simulink model "Crazyflie_angular_velocity_control_PID"  (R2020b)
settings: Solver=VariableStepAuto  StartTime=0.0  StopTime=5  RelTol=1e-3
libraries: pid_lib x4
settings Model: Creator=kt012  LastModifiedBy=kt012

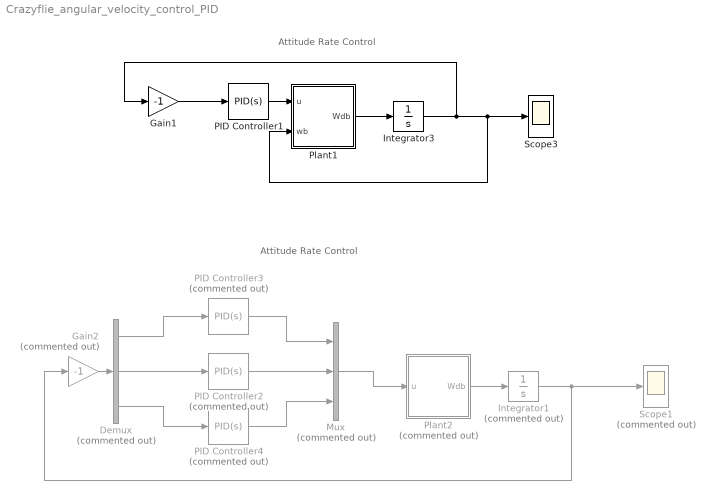
== system Crazyflie_angular_velocity_control_PID ==
  note: Attitude Rate Control
  note: Attitude Rate Control
  Demux : Demux  Commented=on  Outputs=3
  Gain1 : Gain  Gain=-1
  Gain2 : Gain  Commented=on  Gain=-1
  Integrator1 : Integrator  Commented=on  InitialCondition=[1 0 0];  ContinuousStateAttributes='Wb'
  Integrator3 : Integrator  InitialCondition=[1 0 0];  ContinuousStateAttributes='Wb'
  Mux : Mux  Commented=on  Inputs=3
  PID Controller1 : pid_lib/PID Controller  Controller=PID  Form=Parallel  TimeDomain=Continuous-time  UseExternalTs=off  SampleTime=-1  IntegratorMethod=Forward Euler  FilterMethod=Forward Euler  ControllerParametersSource=internal  P=2500  I=90  D=25  UseFilter=on  N=100  TunerSelectOption=Transfer Function Based (PID Tuner App)  InitialConditionSource=internal  InitialConditionForIntegrator=0  InitialConditionForFilter=0  DifferentiatorICPrevScaledInput=0  ExternalReset=none  TrackingMode=off  Kt=1  LimitOutput=off  SatLimitsSource=internal  UpperSaturationLimit=inf  LowerSaturationLimit=-inf  LinearizeAsGain=on  AntiWindupMode=none  Kb=1  POutMin=[]  POutMax=[]  IOutMin=[]  IOutMax=[]  DOutMin=[]  DOutMax=[]  NOutMin=[]  NOutMax=[]  SumOutMin=[]  SumOutMax=[]  SaturationOutMin=[]  SaturationOutMax=[]  PParamMin=[]  PParamMax=[]  IParamMin=[]  IParamMax=[]  DParamMin=[]  DParamMax=[]  NParamMin=[]  NParamMax=[]  KbParamMin=[]  KbParamMax=[]  KtParamMin=[]  KtParamMax=[]  KbOutMin=[]  KbOutMax=[]  KtOutMin=[]  KtOutMax=[]  IntegratorOutMin=[]  IntegratorOutMax=[]  FilterOutMin=[]  FilterOutMax=[]  SumI1OutMin=[]  SumI1OutMax=[]  SumI2OutMin=[]  SumI2OutMax=[]  SumI3OutMin=[]  SumI3OutMax=[]  SumI4OutMin=[]  SumI4OutMax=[]  SumDOutMin=[]  SumDOutMax=[]  DifferentiatorOutMin=[]  DifferentiatorOutMax=[]  FilterDiffOutCoefMin=[]  FilterDiffOutCoefMax=[]  ReciprocalOutMin=[]  ReciprocalOutMax=[]  SumDenOutMin=[]  SumDenOutMax=[]  SumNumOutMin=[]  SumNumOutMax=[]  DivideOutMin=[]  DivideOutMax=[]  UdiffTsProdOutMin=[]  UdiffTsProdOutMax=[]  NTsProdOutMin=[]  NTsProdOutMax=[]  UintegralTsProdOutMin=[]  UintegralTsProdOutMax=[]  UngainTsProdOutMin=[]  UngainTsProdOutMax=[]  IntegratorContinuousStateAttributes=''  IntegratorStateMustResolveToSignalObject=off  IntegratorRTWStateStorageClass=Auto  FilterContinuousStateAttributes=''  FilterStateMustResolveToSignalObject=off  FilterRTWStateStorageClass=Auto  ParallelPVariant=InternalParameters  IdealPVariant=Disabled  IVariant=InternalParameters  DVariant=InternalParameters  IntegratorVariant=Continuous  SatVariant=Disabled  AWVariant=Passthrough  PCopyVariant=Disabled  TRVariant=Disabled  FdbkBlocksVariant=Forward  IdealPFdbkVariant=Disabled  SatFdbkVariant=Disabled  DerivativeFilterVariant=ContFilter  NVariant=InternalParameters  NCopyVariant=Disabled  FilterICVariant=InternalICsFilter  IntegratorICVariant=InternalICs  ExternalResetVariant=Disabled  TRSumVariant=Passthrough  SumFdbkVariant=Disabled  SumVariant=Sum_PID  TsampFilterVariant=InternalTs  TsampNgainVariant=Passthrough  TsampIntegralVariant=Passthrough  ExternalSaturationOutDataTypeStr=Inherit: Same as second input
  PID Controller2 : pid_lib/PID Controller  Commented=on  Controller=PID  Form=Parallel  TimeDomain=Continuous-time  UseExternalTs=off  SampleTime=-1  IntegratorMethod=Forward Euler  FilterMethod=Forward Euler  ControllerParametersSource=internal  P=2500  I=90  D=25  UseFilter=on  N=100  TunerSelectOption=Transfer Function Based (PID Tuner App)  InitialConditionSource=internal  InitialConditionForIntegrator=0  InitialConditionForFilter=0  DifferentiatorICPrevScaledInput=0  ExternalReset=none  TrackingMode=off  Kt=1  LimitOutput=off  SatLimitsSource=internal  UpperSaturationLimit=inf  LowerSaturationLimit=-inf  LinearizeAsGain=on  AntiWindupMode=none  Kb=1  POutMin=[]  POutMax=[]  IOutMin=[]  IOutMax=[]  DOutMin=[]  DOutMax=[]  NOutMin=[]  NOutMax=[]  SumOutMin=[]  SumOutMax=[]  SaturationOutMin=[]  SaturationOutMax=[]  PParamMin=[]  PParamMax=[]  IParamMin=[]  IParamMax=[]  DParamMin=[]  DParamMax=[]  NParamMin=[]  NParamMax=[]  KbParamMin=[]  KbParamMax=[]  KtParamMin=[]  KtParamMax=[]  KbOutMin=[]  KbOutMax=[]  KtOutMin=[]  KtOutMax=[]  IntegratorOutMin=[]  IntegratorOutMax=[]  FilterOutMin=[]  FilterOutMax=[]  SumI1OutMin=[]  SumI1OutMax=[]  SumI2OutMin=[]  SumI2OutMax=[]  SumI3OutMin=[]  SumI3OutMax=[]  SumI4OutMin=[]  SumI4OutMax=[]  SumDOutMin=[]  SumDOutMax=[]  DifferentiatorOutMin=[]  DifferentiatorOutMax=[]  FilterDiffOutCoefMin=[]  FilterDiffOutCoefMax=[]  ReciprocalOutMin=[]  ReciprocalOutMax=[]  SumDenOutMin=[]  SumDenOutMax=[]  SumNumOutMin=[]  SumNumOutMax=[]  DivideOutMin=[]  DivideOutMax=[]  UdiffTsProdOutMin=[]  UdiffTsProdOutMax=[]  NTsProdOutMin=[]  NTsProdOutMax=[]  UintegralTsProdOutMin=[]  UintegralTsProdOutMax=[]  UngainTsProdOutMin=[]  UngainTsProdOutMax=[]  IntegratorContinuousStateAttributes=''  IntegratorStateMustResolveToSignalObject=off  IntegratorRTWStateStorageClass=Auto  FilterContinuousStateAttributes=''  FilterStateMustResolveToSignalObject=off  FilterRTWStateStorageClass=Auto  ParallelPVariant=InternalParameters  IdealPVariant=Disabled  IVariant=InternalParameters  DVariant=InternalParameters  IntegratorVariant=Continuous  SatVariant=Disabled  AWVariant=Passthrough  PCopyVariant=Disabled  TRVariant=Disabled  FdbkBlocksVariant=Forward  IdealPFdbkVariant=Disabled  SatFdbkVariant=Disabled  DerivativeFilterVariant=ContFilter  NVariant=InternalParameters  NCopyVariant=Disabled  FilterICVariant=InternalICsFilter  IntegratorICVariant=InternalICs  ExternalResetVariant=Disabled  TRSumVariant=Passthrough  SumFdbkVariant=Disabled  SumVariant=Sum_PID  TsampFilterVariant=InternalTs  TsampNgainVariant=Passthrough  TsampIntegralVariant=Passthrough  ExternalSaturationOutDataTypeStr=Inherit: Same as second input
  PID Controller3 : pid_lib/PID Controller  Commented=on  Controller=PID  Form=Parallel  TimeDomain=Continuous-time  UseExternalTs=off  SampleTime=-1  IntegratorMethod=Forward Euler  FilterMethod=Forward Euler  ControllerParametersSource=internal  P=1250  I=2500  D=20  UseFilter=on  N=90.5133762745109  TunerSelectOption=Transfer Function Based (PID Tuner App)  InitialConditionSource=internal  InitialConditionForIntegrator=0  InitialConditionForFilter=0  DifferentiatorICPrevScaledInput=0  ExternalReset=none  TrackingMode=off  Kt=1  LimitOutput=off  SatLimitsSource=internal  UpperSaturationLimit=inf  LowerSaturationLimit=-inf  LinearizeAsGain=on  AntiWindupMode=none  Kb=1  POutMin=[]  POutMax=[]  IOutMin=[]  IOutMax=[]  DOutMin=[]  DOutMax=[]  NOutMin=[]  NOutMax=[]  SumOutMin=[]  SumOutMax=[]  SaturationOutMin=[]  SaturationOutMax=[]  PParamMin=[]  PParamMax=[]  IParamMin=[]  IParamMax=[]  DParamMin=[]  DParamMax=[]  NParamMin=[]  NParamMax=[]  KbParamMin=[]  KbParamMax=[]  KtParamMin=[]  KtParamMax=[]  KbOutMin=[]  KbOutMax=[]  KtOutMin=[]  KtOutMax=[]  IntegratorOutMin=[]  IntegratorOutMax=[]  FilterOutMin=[]  FilterOutMax=[]  SumI1OutMin=[]  SumI1OutMax=[]  SumI2OutMin=[]  SumI2OutMax=[]  SumI3OutMin=[]  SumI3OutMax=[]  SumI4OutMin=[]  SumI4OutMax=[]  SumDOutMin=[]  SumDOutMax=[]  DifferentiatorOutMin=[]  DifferentiatorOutMax=[]  FilterDiffOutCoefMin=[]  FilterDiffOutCoefMax=[]  ReciprocalOutMin=[]  ReciprocalOutMax=[]  SumDenOutMin=[]  SumDenOutMax=[]  SumNumOutMin=[]  SumNumOutMax=[]  DivideOutMin=[]  DivideOutMax=[]  UdiffTsProdOutMin=[]  UdiffTsProdOutMax=[]  NTsProdOutMin=[]  NTsProdOutMax=[]  UintegralTsProdOutMin=[]  UintegralTsProdOutMax=[]  UngainTsProdOutMin=[]  UngainTsProdOutMax=[]  IntegratorContinuousStateAttributes=''  IntegratorStateMustResolveToSignalObject=off  IntegratorRTWStateStorageClass=Auto  FilterContinuousStateAttributes=''  FilterStateMustResolveToSignalObject=off  FilterRTWStateStorageClass=Auto  ParallelPVariant=InternalParameters  IdealPVariant=Disabled  IVariant=InternalParameters  DVariant=InternalParameters  IntegratorVariant=Continuous  SatVariant=Disabled  AWVariant=Passthrough  PCopyVariant=Disabled  TRVariant=Disabled  FdbkBlocksVariant=Forward  IdealPFdbkVariant=Disabled  SatFdbkVariant=Disabled  DerivativeFilterVariant=ContFilter  NVariant=InternalParameters  NCopyVariant=Disabled  FilterICVariant=InternalICsFilter  IntegratorICVariant=InternalICs  ExternalResetVariant=Disabled  TRSumVariant=Passthrough  SumFdbkVariant=Disabled  SumVariant=Sum_PID  TsampFilterVariant=InternalTs  TsampNgainVariant=Passthrough  TsampIntegralVariant=Passthrough  ExternalSaturationOutDataTypeStr=Inherit: Same as second input
  PID Controller4 : pid_lib/PID Controller  Commented=on  Controller=PID  Form=Parallel  TimeDomain=Continuous-time  UseExternalTs=off  SampleTime=-1  IntegratorMethod=Forward Euler  FilterMethod=Forward Euler  ControllerParametersSource=internal  P=2500  I=90  D=25  UseFilter=on  N=100  TunerSelectOption=Transfer Function Based (PID Tuner App)  InitialConditionSource=internal  InitialConditionForIntegrator=0  InitialConditionForFilter=0  DifferentiatorICPrevScaledInput=0  ExternalReset=none  TrackingMode=off  Kt=1  LimitOutput=off  SatLimitsSource=internal  UpperSaturationLimit=inf  LowerSaturationLimit=-inf  LinearizeAsGain=on  AntiWindupMode=none  Kb=1  POutMin=[]  POutMax=[]  IOutMin=[]  IOutMax=[]  DOutMin=[]  DOutMax=[]  NOutMin=[]  NOutMax=[]  SumOutMin=[]  SumOutMax=[]  SaturationOutMin=[]  SaturationOutMax=[]  PParamMin=[]  PParamMax=[]  IParamMin=[]  IParamMax=[]  DParamMin=[]  DParamMax=[]  NParamMin=[]  NParamMax=[]  KbParamMin=[]  KbParamMax=[]  KtParamMin=[]  KtParamMax=[]  KbOutMin=[]  KbOutMax=[]  KtOutMin=[]  KtOutMax=[]  IntegratorOutMin=[]  IntegratorOutMax=[]  FilterOutMin=[]  FilterOutMax=[]  SumI1OutMin=[]  SumI1OutMax=[]  SumI2OutMin=[]  SumI2OutMax=[]  SumI3OutMin=[]  SumI3OutMax=[]  SumI4OutMin=[]  SumI4OutMax=[]  SumDOutMin=[]  SumDOutMax=[]  DifferentiatorOutMin=[]  DifferentiatorOutMax=[]  FilterDiffOutCoefMin=[]  FilterDiffOutCoefMax=[]  ReciprocalOutMin=[]  ReciprocalOutMax=[]  SumDenOutMin=[]  SumDenOutMax=[]  SumNumOutMin=[]  SumNumOutMax=[]  DivideOutMin=[]  DivideOutMax=[]  UdiffTsProdOutMin=[]  UdiffTsProdOutMax=[]  NTsProdOutMin=[]  NTsProdOutMax=[]  UintegralTsProdOutMin=[]  UintegralTsProdOutMax=[]  UngainTsProdOutMin=[]  UngainTsProdOutMax=[]  IntegratorContinuousStateAttributes=''  IntegratorStateMustResolveToSignalObject=off  IntegratorRTWStateStorageClass=Auto  FilterContinuousStateAttributes=''  FilterStateMustResolveToSignalObject=off  FilterRTWStateStorageClass=Auto  ParallelPVariant=InternalParameters  IdealPVariant=Disabled  IVariant=InternalParameters  DVariant=InternalParameters  IntegratorVariant=Continuous  SatVariant=Disabled  AWVariant=Passthrough  PCopyVariant=Disabled  TRVariant=Disabled  FdbkBlocksVariant=Forward  IdealPFdbkVariant=Disabled  SatFdbkVariant=Disabled  DerivativeFilterVariant=ContFilter  NVariant=InternalParameters  NCopyVariant=Disabled  FilterICVariant=InternalICsFilter  IntegratorICVariant=InternalICs  ExternalResetVariant=Disabled  TRSumVariant=Passthrough  SumFdbkVariant=Disabled  SumVariant=Sum_PID  TsampFilterVariant=InternalTs  TsampNgainVariant=Passthrough  TsampIntegralVariant=Passthrough  ExternalSaturationOutDataTypeStr=Inherit: Same as second input
  Plant1 : Subsystem
  Plant2 : Subsystem  Commented=on
  Scope1 : Scope  Commented=on
  Scope3 : Scope
  wires:
  PID Controller1/1 -> Plant1/1(u)
  Plant1/1(Wdb) -> Integrator3/1
  Gain1/1 -> PID Controller1/1
  Integrator3/1 -> Gain1/1, Plant1/2(wb), Scope3/1
  PID Controller2/1 -> Mux/2
  Integrator1/1 -> Gain2/1, Scope1/1
  Gain2/1 -> Demux/1
  Plant2/1(Wdb) -> Integrator1/1
  Demux/1 -> PID Controller3/1
  Demux/2 -> PID Controller2/1
  Demux/3 -> PID Controller4/1
  PID Controller4/1 -> Mux/3
  PID Controller3/1 -> Mux/1
  Mux/1 -> Plant2/1(u)

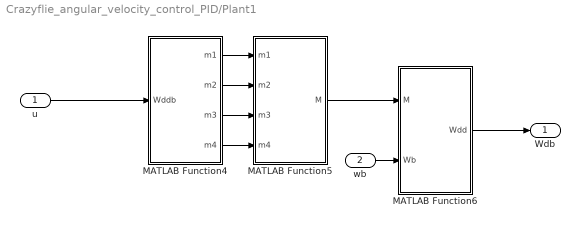
== system Crazyflie_angular_velocity_control_PID/Plant1 ==
  u : Inport
  wb : Inport  Port=2
  MATLAB Function4 : MATLAB Function  TreatAsAtomicUnit=on
  MATLAB Function5 : MATLAB Function  TreatAsAtomicUnit=on
  MATLAB Function6 : MATLAB Function  TreatAsAtomicUnit=on
  Wdb : Outport
  wires:
  wb/1 -> MATLAB Function6/2(Wb)
  MATLAB Function5/1(M) -> MATLAB Function6/1(M)
  MATLAB Function6/1(Wdd) -> Wdb/1
  MATLAB Function4/3(m3) -> MATLAB Function5/3(m3)
  MATLAB Function4/2(m2) -> MATLAB Function5/2(m2)
  MATLAB Function4/4(m4) -> MATLAB Function5/4(m4)
  u/1 -> MATLAB Function4/1(Wddb)
  MATLAB Function4/1(m1) -> MATLAB Function5/1(m1)

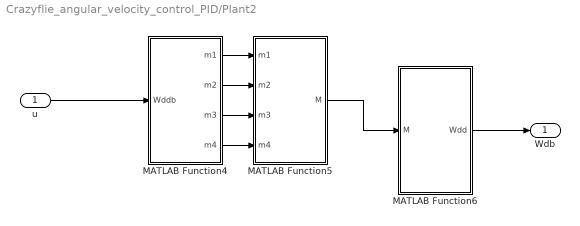
== system Crazyflie_angular_velocity_control_PID/Plant2 ==
  u : Inport
  MATLAB Function4 : MATLAB Function  TreatAsAtomicUnit=on
  MATLAB Function5 : MATLAB Function  TreatAsAtomicUnit=on
  MATLAB Function6 : MATLAB Function  TreatAsAtomicUnit=on
  Wdb : Outport
  wires:
  MATLAB Function5/1(M) -> MATLAB Function6/1(M)
  MATLAB Function6/1(Wdd) -> Wdb/1
  MATLAB Function4/3(m3) -> MATLAB Function5/3(m3)
  MATLAB Function4/2(m2) -> MATLAB Function5/2(m2)
  MATLAB Function4/4(m4) -> MATLAB Function5/4(m4)
  u/1 -> MATLAB Function4/1(Wddb)
  MATLAB Function4/1(m1) -> MATLAB Function5/1(m1)

== matlab function Crazyflie_angular_velocity_control_PID/Plant1/MATLAB Function4 ==
  data: Wddb input; m1 output; m2 output; m3 output; m4 output
function [m1, m2, m3, m4]= fcn(Wddb)

% F [16bit] Wddb [16bit]

r = min(max(-32000, Wddb(1)), 32000)/2;
p = min(max(-32000, Wddb(2)), 32000)/2;
y = min(max(-32000, Wddb(3)), 32000);

m1 = min(max(0, - r - p + y), 2^16);
m2 = min(max(0, - r + p - y), 2^16);
m3 = min(max(0, + r + p + y), 2^16);
m4 = min(max(0, + r - p - y), 2^16);

% formation +
% r = min(max(-32000, Wddb(1)), 32000);
% p = min(max(-32000, Wddb(2)), 32000);
% y = min(max(-32000, Wddb(3)), 32000);
% m1 = min(max(0, + p + y), 2^16);
% m2 = min(max(0, - r - y), 2^16);
% m3 = min(max(0, - p + y), 2^16);
% m4 = min(max(0, + r - y), 2^16);

%         ^y
%         |
%         |
%   m3          m4
%
%                    ------>x
%
%   m2          m1

== matlab function Crazyflie_angular_velocity_control_PID/Plant2/MATLAB Function4 ==
  data: Wddb input; m1 output; m2 output; m3 output; m4 output
function [m1, m2, m3, m4]= fcn(Wddb)

% F [16bit] Wddb [16bit]

r = min(max(-32000, Wddb(1)), 32000)/2;
p = min(max(-32000, Wddb(2)), 32000)/2;
y = min(max(-32000, Wddb(3)), 32000);

m1 = min(max(0, - r - p + y), 2^16);
m2 = min(max(0, - r + p - y), 2^16);
m3 = min(max(0, + r + p + y), 2^16);
m4 = min(max(0, + r - p - y), 2^16);

% formation +
% r = min(max(-32000, Wddb(1)), 32000);
% p = min(max(-32000, Wddb(2)), 32000);
% y = min(max(-32000, Wddb(3)), 32000);
% m1 = min(max(0, + p + y), 2^16);
% m2 = min(max(0, - r - y), 2^16);
% m3 = min(max(0, - p + y), 2^16);
% m4 = min(max(0, + r - y), 2^16);

%         ^y
%         |
%         |
%   m3          m4
%
%                    ------>x
%
%   m2          m1

== matlab function Crazyflie_angular_velocity_control_PID/Plant2/MATLAB Function5 ==
  data: m1 input; m2 input; M output; m3 input; m4 input
function M = func(m1, m2, m3, m4)

% F [16bit] Wddb [16bit]
g = 9.8;
Armlength = 0.092/2;
Armlength = 0.092/2;
m1 = 2.130295 * 10^(-11) * m1^2 +  1.032633 * 10^(-6) * m1 + 5.484560 * 10^(-4);
m2 = 2.130295 * 10^(-11) * m2^2 +  1.032633 * 10^(-6) * m2 + 5.484560 * 10^(-4);
m3 = 2.130295 * 10^(-11) * m3^2 +  1.032633 * 10^(-6) * m3 + 5.484560 * 10^(-4);
m4 = 2.130295 * 10^(-11) * m4^2 +  1.032633 * 10^(-6) * m4 + 5.484560 * 10^(-4);

% formation X
M1 = Armlength / sqrt(2) * (m3 + m4 - m1 - m2);
M2 = -Armlength / sqrt(2) * (-m3 - m2 + m1 + m4);

% formation + 
% M1 = Armlength  * (m4 - m2);
% M2 = Armlength * (m1 - m3);

M3 = m1 + m3 - m2 - m4;
M = [M1 M2 M3]';

== matlab function Crazyflie_angular_velocity_control_PID/Plant1/MATLAB Function5 ==
  data: m1 input; m2 input; M output; m3 input; m4 input
function M = func(m1, m2, m3, m4)

% F [16bit] Wddb [16bit]
g = 9.8;
Armlength = 0.092/2;
Armlength = 0.092/2;
m1 = 2.130295 * 10^(-11) * m1^2 +  1.032633 * 10^(-6) * m1 + 5.484560 * 10^(-4);
m2 = 2.130295 * 10^(-11) * m2^2 +  1.032633 * 10^(-6) * m2 + 5.484560 * 10^(-4);
m3 = 2.130295 * 10^(-11) * m3^2 +  1.032633 * 10^(-6) * m3 + 5.484560 * 10^(-4);
m4 = 2.130295 * 10^(-11) * m4^2 +  1.032633 * 10^(-6) * m4 + 5.484560 * 10^(-4);

% formation X
M1 = Armlength / sqrt(2) * (m3 + m4 - m1 - m2);
M2 = -Armlength / sqrt(2) * (-m3 - m2 + m1 + m4);

% formation + 
% M1 = Armlength  * (m4 - m2);
% M2 = Armlength * (m1 - m3);

M3 = m1 + m3 - m2 - m4;
M = [M1 M2 M3]';

== matlab function Crazyflie_angular_velocity_control_PID/Plant1/MATLAB Function6 ==
  data: M input; Wb input; Wdd output
function Wdd = fcn(M,Wb)

% % crazyflie
I = [16.571710 0.830806 0.718277;
     0.830806 16.655602 1.800197;
     0.718277 1.800197 29.261652] * 10^(-6);      % crazyflieの慣性モーメント（kg・m^2）
I = [1 0 0;
     0 1 0;
     0 0 1] * 10^(-6);
% 各加速度計算（ボディー座標系）
Wdd = pinv(I)*(M - cross(Wb, I * Wb));

== matlab function Crazyflie_angular_velocity_control_PID/Plant2/MATLAB Function6 ==
  data: M input; Wdd output
function Wdd = fcn(M)

% % crazyflie
I = [16.571710 0.830806 0.718277;
     0.830806 16.655602 1.800197;
     0.718277 1.800197 29.261652] * 10^(-6);      % crazyflieの慣性モーメント（kg・m^2）
I = [1 0 0;
     0 1 0;
     0 0 1] * 10^(-6);
% 各加速度計算（ボディー座標系）
Wdd = 10^(-6) * M;
